simulink model "ArduinoBase"  (R2022b)
settings: Solver=ode2  StartTime=0.0  StopTime=inf  FixedStep=0.01  RelTol=1e-3  EnableMultiTasking=on
undefined symbols (not defined in the file): ODR
libraries: arduinosensorlib x2, cstblocks x1
settings Model: ExtModeTrigDuration=2  Creator=raul  LastModifiedBy=raul
settings OptimizationCC: EnhancedBackFolding=on  PassReuseOutputArgsAs=Individual arguments  ZeroExternalMemoryAtStartup=off  ZeroInternalMemoryAtStartup=off  MaxStackSize=64  OptimizeBlockOrder=speed  DifferentSizesBufferReuse=on  OptimizationCustomize=off  EfficientTunableParamExpr=on
settings DebuggingCC: ParameterTunabilityLossMsg=error
settings HardwareCC: ProdBitPerInt=16  ProdBitPerPointer=16  ProdBitPerSizeT=16  ProdBitPerPtrDiffT=16  ProdLargestAtomicFloat=None  ProdWordSize=8  ProdHWDeviceType=Atmel->AVR  UseEmbeddedCoderFeatures=off  UseSimulinkCoderFeatures=off
settings SFSimCC: MATLABDynamicMemAlloc=off
settings RTWCC: Description=Embedded Coder  SystemTargetFile=ert.tlc  HardwareBoard=Arduino Uno  TLCOptions=-aInlineSetEventsForThisBaseRateFcn=TLC_FALSE -aSuppressMultiTaskScheduler=TLC_FALSE -aRateBasedStepFcn=1  TemplateMakefile=ert_default_tmf  Toolchain=Arduino AVR  BuildConfiguration=Faster Runs
settings CodeAppCC: ForceParamTrailComments=on  IgnoreCustomStorageClasses=off  OperatorAnnotations=on  SimulinkDataObjDesc=on  SFDataObjDesc=on  InsertBlockDesc=on
settings ERTTargetCC: SupportContinuousTime=on  SupportNonInlinedSFcns=on  SupportVariableSizeSignals=on  ExtModeTransport=3  ExtModeStaticAlloc=on  ExtModeAutomaticAllocSize=off  ExtModeStaticAllocSize=250  ExtModeMexFile=ext_xcp  ExtModeIntrfLevel=Level2 - Open

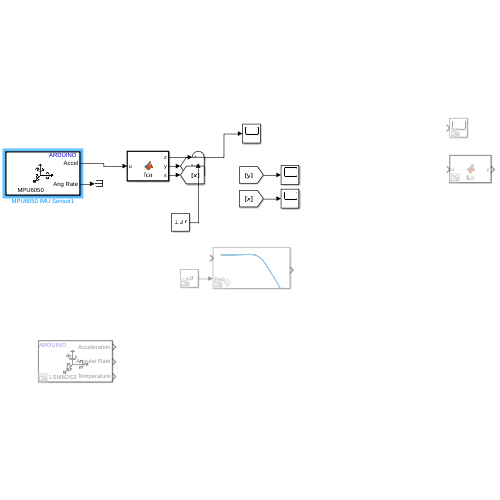
[thumbnail: Simulink's stored preview of the top-level diagram]
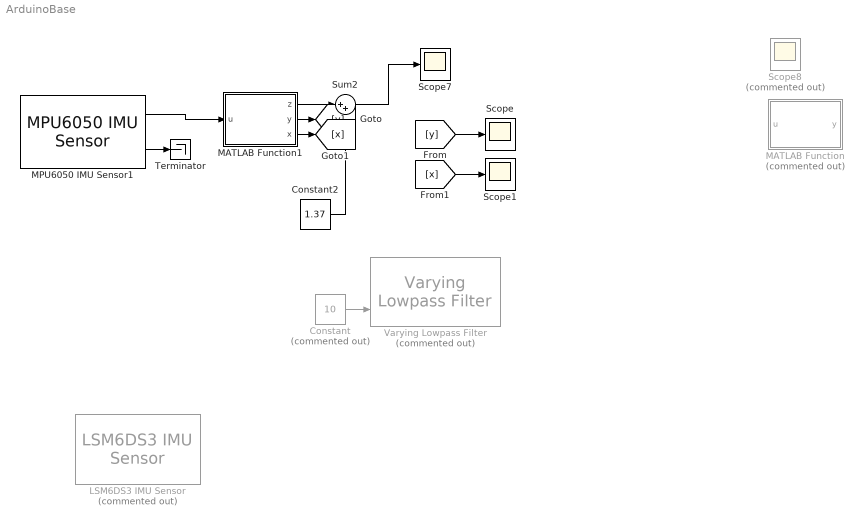
== system ArduinoBase ==
  Constant : Constant  Commented=on  Value=10
  Constant2 : Constant  Value=1.37
  LSM6DS3 IMU Sensor : arduinosensorlib/LSM6DS3 IMU Sensor  Commented=on  I2CAddress=0x6A  IsActiveAcceleration=on  IsActiveAngularRate=on  IsActiveTemperature=on  IsActiveStatus=off  IsActiveTimeStamp=off  spf=1  SampleTime=-1  QueueSizeFactor=1  AccelerometerRange=+/- 2g  AccelerometerODR=12.5 Hz  SelectAnalogBW=off  AccelLPF1BW=400 Hz  AccelSelectCompositeFilter=No filter  AccelLPF2BW=ODR/50  AccelHPFBW=ODR/100  GyroscopeRange=250 dps  GyroscopeODR=12.5 Hz  SelectGyroscopeHPF=off  GyroHPFBW=0.0081 Hz
  MATLAB Function : MATLAB Function  Commented=on  TreatAsAtomicUnit=on
  MATLAB Function1 : MATLAB Function  TreatAsAtomicUnit=on
  MPU6050 IMU Sensor1 : arduinosensorlib/MPU6050 IMU Sensor  SlaveAddress=0x68  Accel=on  AngularRate=on  Temperature=off  Status=off  Timestamp=off  EulerAngles=off  Quat=off  AccelRange=16G  GyroRange=2000 dps  DmpOdr=200 Hz  Dlpf=Accelerometer: 260Hz, Gyroscope: 256Hz  spf=1  SampleTime=-1  QueueSizeFactor=1
  Scope : Scope
  Scope1 : Scope
  Scope7 : Scope
  Scope8 : Scope  Commented=on
  Sum2 : Sum  Inputs=|++
  Terminator : Terminator
  Varying Lowpass Filter : cstblocks/Linear Parameter Varying/Varying Lowpass Filter  Commented=on  N=1
  wires:
  MPU6050 IMU Sensor1/1 -> MATLAB Function1/1(u)
  MPU6050 IMU Sensor1/2 -> Terminator/1
  Constant2/1 -> Sum2/2
  Sum2/1 -> Scope7/1
  Constant/1 -> Varying Lowpass Filter/2
  MATLAB Function1/1(z) -> Sum2/1
  MATLAB Function1/2(y) -> [y]
  MATLAB Function1/3(x) -> [x]
  [y] -> Scope/1
  [x] -> Scope1/1

== matlab function ArduinoBase/MATLAB Function1 ==
  data: z output; u input; y output; x output
function [z,y,x] = fcn(u)

z = u(3,:,:);
y = u(2,:,:);
x = u(1,:,:);

== matlab function ArduinoBase/MATLAB Function ==
  data: u input; y output
function y = fcn(u)

a=0.05;

if u < a || u > -a
    y=0;
else
    y = u;
end
